simulink model "stateFeedback"  (R2024b)
settings: Solver=VariableStepAuto  StartTime=0.0  StopTime=1  RelTol=1e-3
undefined symbols (not defined in the file): A, B, C, K, x_0
settings Model: Creator=Longbin  LastModifiedBy=Longbin

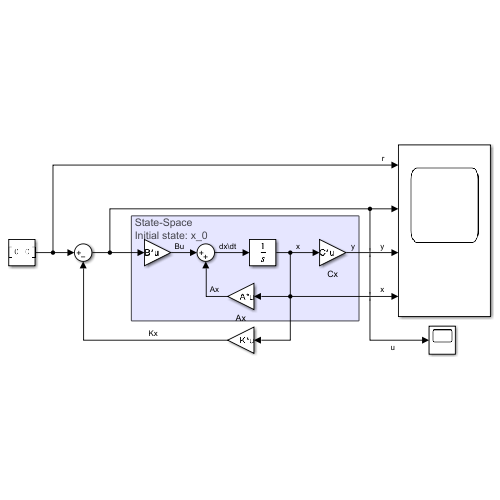
[thumbnail: Simulink's stored preview of the top-level diagram]
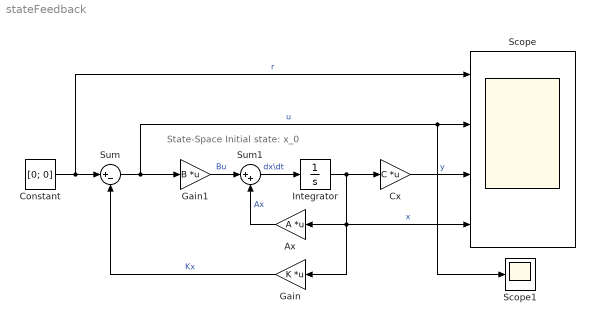
== system stateFeedback ==
  note: State-Space
      | Initial state: x_0
  Ax : Gain  Gain=A  Multiplication=Matrix(K*u)
  Constant : Constant  Value=[0; 0]
  Cx : Gain  Gain=C  Multiplication=Matrix(K*u)
  Gain : Gain  Gain=K  Multiplication=Matrix(K*u)
  Gain1 : Gain  Gain=B  Multiplication=Matrix(K*u)
  Integrator : Integrator  InitialCondition=x_0
  Scope : Scope  NumInputPorts=4
  Scope1 : Scope
  Sum : Sum  Inputs=|+-
  Sum1 : Sum  Inputs=|++
  wires:
  Sum/1 -> Gain1/1, Scope1/1, Scope/2  "u"
  Gain/1 -> Sum/2  "Kx"
  Ax/1 -> Sum1/2  "Ax"
  Gain1/1 -> Sum1/1  "Bu"
  Cx/1 -> Scope/3  "y"
  Sum1/1 -> Integrator/1  "dx\\dt"
  Integrator/1 -> Cx/1, Gain/1, Scope/4, Ax/1  "x"
  Constant/1 -> Scope/1, Sum/1  "r"
